simulink model "sendandrecieve"  (R2016b)
settings: Solver=VariableStepAuto  StartTime=0.0  StopTime=0.01  RelTol=1e-3
undefined symbols (not defined in the file or in its folder): Rec, SDTV
libraries: etargetslib x10, dspnetwork x10, visionconversions x2, visionsources x1
settings Model: Creator=zeabus  LastModifiedBy=zeabus

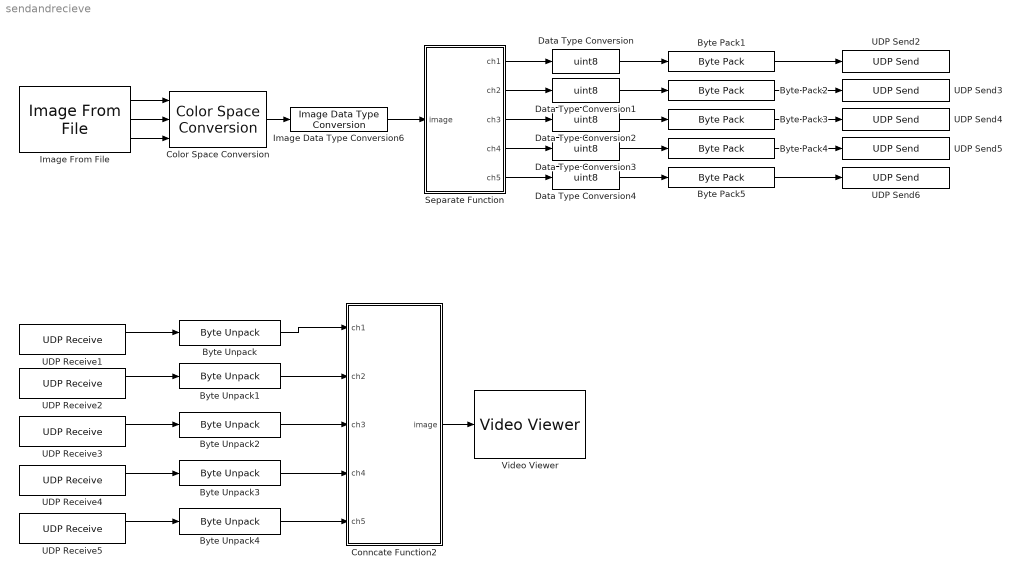
== system sendandrecieve ==
  Byte Pack{1..5} (5 alike) : etargetslib/Byte Pack  datatypes={'uint8'}  byteAlign=1
  Byte Unpack{,1..4} (5 alike) : etargetslib/Byte Unpack  dimensions={[61440]}  datatypes={'uint8'}  byteAlign=1
  Color Space Conversion : visionconversions/Color Space  Conversion  conversion=Obsolete  conversionActive=R'G'B' to intensity  wp_str=D65  rec=Rec. 601 (SDTV)  sys=1125/60/2:1  imagePorts=Separate color signals
  Conncate Function2 : MATLAB Function  TreatAsAtomicUnit=on
  Data Type Conversion{,1..4} (5 alike) : DataTypeConversion  OutDataTypeStr=uint8
  Image Data Type Conversion6 : visionconversions/Image Data Type Conversion  outDT=uint8  isSigned=on  wordLen=16  numFracBits=0
  Image From File : visionsources/Image From File  Tag=vipblks_nd  FileName=C:\Users\zeabus\Desktop\Workspace\matlab\vision\images\640480.fw.png  imagePorts=Separate color signals  Ts=inf  ImageDataType=Inherit from input image  Signed=on  WordLength=16  sdImageDataType=uint(8)  FractionLengthMode=User-defined  FractionLength=15  OutPortLabels=R|G|B
  Separate Function : MATLAB Function  TreatAsAtomicUnit=on
  UDP Receive1 : dspnetwork/UDP Receive  localURL='0.0.0.0'  localPort=30000  remoteURL='0.0.0.0'  remotePort=-1  recvBufferSize=61440  dims=61440  signalDatatype=uint8  isVarSize=off  showBlockingTime=on  blockingTime=0.01  sampletime=0.01  blockPlatform=HOST
  UDP Receive2 : dspnetwork/UDP Receive  localURL='0.0.0.0'  localPort=30001  remoteURL='0.0.0.0'  remotePort=-1  recvBufferSize=61440  dims=61440  signalDatatype=uint8  isVarSize=off  showBlockingTime=on  blockingTime=0.01  sampletime=0.01  blockPlatform=HOST
  UDP Receive3 : dspnetwork/UDP Receive  localURL='0.0.0.0'  localPort=30002  remoteURL='0.0.0.0'  remotePort=-1  recvBufferSize=61440  dims=61440  signalDatatype=uint8  isVarSize=off  showBlockingTime=on  blockingTime=0.01  sampletime=0.01  blockPlatform=HOST
  UDP Receive4 : dspnetwork/UDP Receive  localURL='0.0.0.0'  localPort=30003  remoteURL='0.0.0.0'  remotePort=-1  recvBufferSize=61440  dims=61440  signalDatatype=uint8  isVarSize=off  showBlockingTime=on  blockingTime=0.01  sampletime=0.01  blockPlatform=HOST
  UDP Receive5 : dspnetwork/UDP Receive  localURL='0.0.0.0'  localPort=30004  remoteURL='0.0.0.0'  remotePort=-1  recvBufferSize=61440  dims=61440  signalDatatype=uint8  isVarSize=off  showBlockingTime=on  blockingTime=0.01  sampletime=0.01  blockPlatform=HOST
  UDP Send2 : dspnetwork/UDP Send  remoteURL='255.255.255.255'  remotePort=30000  localURL='0.0.0.0'  localPortSource=Automatically determine  localPort=-1  sampletime=-1  blockPlatform=HOST  separateLengthPort=0
  UDP Send3 : dspnetwork/UDP Send  remoteURL='255.255.255.255'  remotePort=30001  localURL='0.0.0.0'  localPortSource=Automatically determine  localPort=-1  sampletime=-1  blockPlatform=HOST  separateLengthPort=0
  UDP Send4 : dspnetwork/UDP Send  remoteURL='255.255.255.255'  remotePort=30002  localURL='0.0.0.0'  localPortSource=Automatically determine  localPort=-1  sampletime=-1  blockPlatform=HOST  separateLengthPort=0
  UDP Send5 : dspnetwork/UDP Send  remoteURL='255.255.255.255'  remotePort=30003  localURL='0.0.0.0'  localPortSource=Automatically determine  localPort=-1  sampletime=-1  blockPlatform=HOST  separateLengthPort=0
  UDP Send6 : dspnetwork/UDP Send  remoteURL='255.255.255.255'  remotePort=30004  localURL='0.0.0.0'  localPortSource=Automatically determine  localPort=-1  sampletime=-1  blockPlatform=HOST  separateLengthPort=0
  Video Viewer : VideoViewer
  wires:
  UDP Receive1/1 -> Byte Unpack/1
  Image From File/1 -> Color Space Conversion/1
  Image From File/2 -> Color Space Conversion/2
  Image From File/3 -> Color Space Conversion/3
  Image Data Type Conversion6/1 -> Separate Function/1(image)
  Color Space Conversion/1 -> Image Data Type Conversion6/1
  Separate Function/1(ch1) -> Data Type Conversion/1
  Separate Function/2(ch2) -> Data Type Conversion1/1
  Separate Function/4(ch4) -> Data Type Conversion3/1
  Separate Function/3(ch3) -> Data Type Conversion2/1
  Separate Function/5(ch5) -> Data Type Conversion4/1
  Data Type Conversion/1 -> Byte Pack1/1
  Data Type Conversion1/1 -> Byte Pack2/1
  Data Type Conversion2/1 -> Byte Pack3/1
  Data Type Conversion3/1 -> Byte Pack4/1
  Data Type Conversion4/1 -> Byte Pack5/1
  Byte Pack1/1 -> UDP Send2/1
  Byte Pack2/1 -> UDP Send3/1
  Byte Pack3/1 -> UDP Send4/1
  Byte Pack4/1 -> UDP Send5/1
  Byte Pack5/1 -> UDP Send6/1
  UDP Receive2/1 -> Byte Unpack1/1
  UDP Receive3/1 -> Byte Unpack2/1
  UDP Receive4/1 -> Byte Unpack3/1
  UDP Receive5/1 -> Byte Unpack4/1
  Byte Unpack3/1 -> Conncate Function2/4(ch4)
  Byte Unpack4/1 -> Conncate Function2/5(ch5)
  Byte Unpack2/1 -> Conncate Function2/3(ch3)
  Byte Unpack1/1 -> Conncate Function2/2(ch2)
  Byte Unpack/1 -> Conncate Function2/1(ch1)
  Conncate Function2/1(image) -> Video Viewer/1

== matlab function sendandrecieve/Conncate Function2 ==
  data: ch1 input; ch2 input size=61440; ch3 input size=61440; ch4 input size=61440; ch5 input uint8; image output
function image  = concatenation(ch1,ch2,ch3,ch4,ch5)
maxcol = 128;
height = 480;
width = 640;

ch1 = reshape(ch1,height,maxcol);
ch2 = reshape(ch2,height,maxcol);
ch3 = reshape(ch3,height,maxcol);
ch4 = reshape(ch4,height,maxcol);
ch5 = reshape(ch5,height,maxcol);
image = [ch1,ch2,ch3,ch4,ch5];
image = reshape(image,height,width);

== matlab function sendandrecieve/Separate Function ==
  data: image input; ch1 output; ch2 output; ch3 output; ch4 output; ch5 output
function [ch1,ch2,ch3,ch4,ch5] = separate(image)
maxlength = 307200;
dividelength = 61440;

image = reshape(image,1,maxlength);
ch1 = image(1:dividelength);
ch2 = image(dividelength*1+1:dividelength*2);
ch3 = image(dividelength*2+1:dividelength*3);
ch4 = image(dividelength*3+1:dividelength*4);
ch5 = image(dividelength*4+1:dividelength*5);
